simulink model "AFlutter"  (Simulink 7.7)
settings: Solver=FixedStepDiscrete  StartTime=0.0  StopTime=1000000  FixedStep=1  RelTol=1e-3
libraries: LookupModeling x68
settings Model: Creator=iris  LastModifiedBy=iris

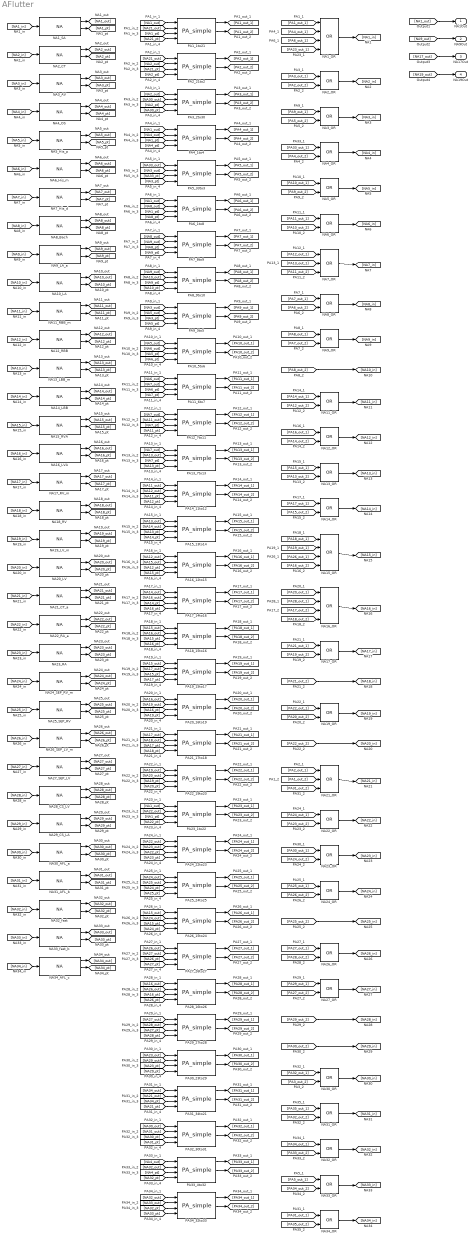
== system AFlutter ==
  NA10_LA : LookupModeling/NA  SystemSampleTime=-1  TERP_s_m=360  TERP_defs_m=360  TRRP_s_m=120  TRRP_def_m=120  Trest_s_m=9999  Trest_def_m=9999  Terp_min_m=150  Terp_max_m=360
  NA11_OR : Logic  Operator=OR  AllPortsSameDT=off  OutDataTypeStr=boolean
  NA11_RBB_m : LookupModeling/NA  SystemSampleTime=-1  TERP_s_m=440  TERP_defs_m=440  TRRP_s_m=120  TRRP_def_m=120  Trest_s_m=9999  Trest_def_m=9999  Terp_min_m=330  Terp_max_m=440
  NA12_OR : Logic  Operator=OR  AllPortsSameDT=off  OutDataTypeStr=boolean
  NA12_RBB : LookupModeling/NA  SystemSampleTime=-1  TERP_s_m=440  TERP_defs_m=440  TRRP_s_m=120  TRRP_def_m=120  Trest_s_m=9999  Trest_def_m=9999  Terp_min_m=330  Terp_max_m=440
  NA13_LBB_m : LookupModeling/NA  SystemSampleTime=-1  TERP_s_m=440  TERP_defs_m=440  TRRP_s_m=120  TRRP_def_m=120  Trest_s_m=9999  Trest_def_m=9999  Terp_min_m=330  Terp_max_m=440
  NA13_OR : Logic  Operator=OR  AllPortsSameDT=off  OutDataTypeStr=boolean
  NA14_LBB : LookupModeling/NA  SystemSampleTime=-1  TERP_s_m=440  TERP_defs_m=440  TRRP_s_m=120  TRRP_def_m=120  Trest_s_m=9999  Trest_def_m=9999  Terp_min_m=330  Terp_max_m=440
  NA14_OR : Logic  Operator=OR  AllPortsSameDT=off  OutDataTypeStr=boolean
  NA15_OR : Logic  Operator=OR  Inputs=4  AllPortsSameDT=off  OutDataTypeStr=boolean
  NA15_RVA : LookupModeling/NA  SystemSampleTime=-1  TERP_s_m=290  TERP_defs_m=290  TRRP_s_m=120  TRRP_def_m=120  Trest_s_m=9999  Trest_def_m=9999  Terp_min_m=180  Terp_max_m=290
  NA16_LVA : LookupModeling/NA  SystemSampleTime=-1  TERP_s_m=290  TERP_defs_m=290  TRRP_s_m=120  TRRP_def_m=120  Trest_s_m=9999  Trest_def_m=9999  Terp_min_m=180  Terp_max_m=290
  NA16_OR : Logic  Operator=OR  Inputs=4  AllPortsSameDT=off  OutDataTypeStr=boolean
  NA17_OR : Logic  Operator=OR  AllPortsSameDT=off  OutDataTypeStr=boolean
  NA17_RV_m : LookupModeling/NA  SystemSampleTime=-1  TERP_s_m=290  TERP_defs_m=290  TRRP_s_m=120  TRRP_def_m=120  Trest_s_m=9999  Trest_def_m=9999  Terp_min_m=180  Terp_max_m=290
  NA18_RV : LookupModeling/NA  SystemSampleTime=-1  TERP_s_m=290  TERP_defs_m=290  TRRP_s_m=120  TRRP_def_m=120  Trest_s_m=9999  Trest_def_m=9999  Terp_min_m=180  Terp_max_m=290
  NA19_LV_m : LookupModeling/NA  SystemSampleTime=-1  TERP_s_m=303  TERP_defs_m=290  TRRP_s_m=120  TRRP_def_m=120  Trest_s_m=9999  Trest_def_m=9999  Terp_min_m=180  Terp_max_m=290
  NA19_OR : Logic  Operator=OR  AllPortsSameDT=off  OutDataTypeStr=boolean
  NA1_OR : Logic  Operator=OR  Inputs=4  AllPortsSameDT=off  OutDataTypeStr=boolean
  NA1_SA : LookupModeling/NA  SystemSampleTime=-1  TERP_s_m=150  TERP_defs_m=150  TRRP_s_m=20  TRRP_def_m=20  Trest_s_m=500  Trest_def_m=700  Terp_min_m=150  Terp_max_m=300
  NA20_LV : LookupModeling/NA  SystemSampleTime=-1  TERP_s_m=290  TERP_defs_m=290  TRRP_s_m=120  TRRP_def_m=120  Trest_s_m=9999  Trest_def_m=9999  Terp_min_m=180  Terp_max_m=290
  NA21_CT_a : LookupModeling/NA  SystemSampleTime=-1  TERP_s_m=180  TERP_defs_m=180  TRRP_s_m=120  TRRP_def_m=120  Trest_s_m=9999  Trest_def_m=9999  Terp_min_m=150  Terp_max_m=200
  NA21_OR : Logic  Operator=OR  Inputs=3  AllPortsSameDT=off  OutDataTypeStr=boolean
  NA22_OR : Logic  Operator=OR  AllPortsSameDT=off  OutDataTypeStr=boolean
  NA22_RA_a : LookupModeling/NA  SystemSampleTime=-1  TERP_s_m=360  TERP_defs_m=360  TRRP_s_m=120  TRRP_def_m=120  Trest_s_m=9999  Trest_def_m=9999  Terp_min_m=150  Terp_max_m=360
  NA23_OR : Logic  Operator=OR  AllPortsSameDT=off  OutDataTypeStr=boolean
  NA23_RA : LookupModeling/NA  SystemSampleTime=-1  TERP_s_m=360  TERP_defs_m=360  TRRP_s_m=120  TRRP_def_m=120  Trest_s_m=9999  Trest_def_m=9999  Terp_min_m=150  Terp_max_m=360
  NA24_OR : Logic  Operator=OR  AllPortsSameDT=off  OutDataTypeStr=boolean
  NA24_SEP_RV_m : LookupModeling/NA  SystemSampleTime=-1  TERP_s_m=300  TERP_defs_m=300  TRRP_s_m=120  TRRP_def_m=120  Trest_s_m=9999  Trest_def_m=9999  Terp_min_m=150  Terp_max_m=300
  NA25_SEP_RV : LookupModeling/NA  SystemSampleTime=-1  TERP_s_m=300  TERP_defs_m=300  TRRP_s_m=120  TRRP_def_m=120  Trest_s_m=9999  Trest_def_m=9999  Terp_min_m=150  Terp_max_m=300
  NA26_OR : Logic  Operator=OR  AllPortsSameDT=off  OutDataTypeStr=boolean
  NA26_SEP_LV_m : LookupModeling/NA  SystemSampleTime=-1  TERP_s_m=300  TERP_defs_m=300  TRRP_s_m=120  TRRP_def_m=120  Trest_s_m=9999  Trest_def_m=9999  Terp_min_m=150  Terp_max_m=300
  NA27_OR : Logic  Operator=OR  AllPortsSameDT=off  OutDataTypeStr=boolean
  NA27_SEP_LV : LookupModeling/NA  SystemSampleTime=-1  TERP_s_m=300  TERP_defs_m=300  TRRP_s_m=120  TRRP_def_m=120  Trest_s_m=9999  Trest_def_m=9999  Terp_min_m=150  Terp_max_m=300
  NA28_CS_LV : LookupModeling/NA  SystemSampleTime=-1  TERP_s_m=300  TERP_defs_m=300  TRRP_s_m=120  TRRP_def_m=120  Trest_s_m=9999  Trest_def_m=9999  Terp_min_m=150  Terp_max_m=300
  NA29_CS_LA : LookupModeling/NA  SystemSampleTime=-1  TERP_s_m=300  TERP_defs_m=300  TRRP_s_m=120  TRRP_def_m=120  Trest_s_m=9999  Trest_def_m=9999  Terp_min_m=150  Terp_max_m=300
  NA2_CT : LookupModeling/NA  SystemSampleTime=-1  TERP_s_m=150  TERP_defs_m=150  TRRP_s_m=100  TRRP_def_m=100  Trest_s_m=9999  Trest_def_m=9999  Terp_min_m=50  Terp_max_m=150
  NA2_OR : Logic  Operator=OR  AllPortsSameDT=off  OutDataTypeStr=boolean
  NA30_AFL_a : LookupModeling/NA  SystemSampleTime=-1  TERP_s_m=150  TERP_defs_m=150  TRRP_s_m=100  TRRP_def_m=100  Trest_s_m=9999  Trest_def_m=9999  Terp_min_m=150  Terp_max_m=200
  NA30_OR : Logic  Operator=OR  AllPortsSameDT=off  OutDataTypeStr=boolean
  NA31_AFL_b : LookupModeling/NA  SystemSampleTime=-1  TERP_s_m=150  TERP_defs_m=150  TRRP_s_m=100  TRRP_def_m=100  Trest_s_m=9999  Trest_def_m=9999  Terp_min_m=150  Terp_max_m=200
  NA31_OR : Logic  Operator=OR  AllPortsSameDT=off  OutDataTypeStr=boolean
  NA32_OR : Logic  Operator=OR  AllPortsSameDT=off  OutDataTypeStr=boolean
  NA32_fast : LookupModeling/NA  SystemSampleTime=-1  TERP_s_m=380  TERP_defs_m=380  TRRP_s_m=10  TRRP_def_m=10  Trest_s_m=9999  Trest_def_m=9999  Terp_min_m=500  Terp_max_m=380
  NA33_OR : Logic  Operator=OR  AllPortsSameDT=off  OutDataTypeStr=boolean
  NA33_fast_b : LookupModeling/NA  SystemSampleTime=-1  TERP_s_m=380  TERP_defs_m=380  TRRP_s_m=10  TRRP_def_m=10  Trest_s_m=9999  Trest_def_m=9999  Terp_min_m=500  Terp_max_m=380
  NA34_AFL_c : LookupModeling/NA  SystemSampleTime=-1  TERP_s_m=150  TERP_defs_m=150  TRRP_s_m=100  TRRP_def_m=100  Trest_s_m=9999  Trest_def_m=9999  Terp_min_m=150  Terp_max_m=200
  NA34_OR : Logic  Operator=OR  AllPortsSameDT=off  OutDataTypeStr=boolean
  NA3_AV : LookupModeling/NA  SystemSampleTime=-1  TERP_s_m=230  TERP_defs_m=230  TRRP_s_m=250  TRRP_def_m=250  Trest_s_m=9999  Trest_def_m=9999  Terp_min_m=350  Terp_max_m=230
  NA3_OR : Logic  Operator=OR  AllPortsSameDT=off  OutDataTypeStr=boolean
  NA4_OR : Logic  Operator=OR  AllPortsSameDT=off  OutDataTypeStr=boolean
  NA4_OS : LookupModeling/NA  SystemSampleTime=-1  TERP_s_m=200  TERP_defs_m=200  TRRP_s_m=120  TRRP_def_m=120  Trest_s_m=9999  Trest_def_m=9999  Terp_min_m=100  Terp_max_m=200
  NA5_His_p : LookupModeling/NA  SystemSampleTime=-1  TERP_s_m=440  TERP_defs_m=440  TRRP_s_m=120  TRRP_def_m=120  Trest_s_m=9999  Trest_def_m=9999  Terp_min_m=330  Terp_max_m=440
  NA5_OR : Logic  Operator=OR  AllPortsSameDT=off  OutDataTypeStr=boolean
  NA6_His_m : LookupModeling/NA  SystemSampleTime=-1  TERP_s_m=440  TERP_defs_m=440  TRRP_s_m=120  TRRP_def_m=120  Trest_s_m=9999  Trest_def_m=9999  Terp_min_m=330  Terp_max_m=440
  NA6_OR : Logic  Operator=OR  AllPortsSameDT=off  OutDataTypeStr=boolean
  NA7_His_d : LookupModeling/NA  SystemSampleTime=-1  TERP_s_m=440  TERP_defs_m=440  TRRP_s_m=120  TRRP_def_m=120  Trest_s_m=9999  Trest_def_m=9999  Terp_min_m=330  Terp_max_m=440
  NA7_OR : Logic  Operator=OR  Inputs=3  AllPortsSameDT=off  OutDataTypeStr=boolean
  NA8_Bach : LookupModeling/NA  SystemSampleTime=-1  TERP_s_m=360  TERP_defs_m=360  TRRP_s_m=120  TRRP_def_m=120  Trest_s_m=9999  Trest_def_m=9999  Terp_min_m=150  Terp_max_m=360
  NA8_OR : Logic  Operator=OR  AllPortsSameDT=off  OutDataTypeStr=boolean
  NA9_LA_a : LookupModeling/NA  SystemSampleTime=-1  TERP_s_m=360  TERP_defs_m=360  TRRP_s_m=120  TRRP_def_m=120  Trest_s_m=9999  Trest_def_m=9999  Terp_min_m=150  Terp_max_m=360
  NA9_OR : Logic  Operator=OR  AllPortsSameDT=off  OutDataTypeStr=boolean
  PA10_5to6 : LookupModeling/PA_simple  SystemSampleTime=-1  min_path_par_m=16  bck_param_m=16  forw_param_m=16
  PA11_6to7 : LookupModeling/PA_simple  SystemSampleTime=-1  min_path_par_m=19  bck_param_m=20  forw_param_m=20
  PA12_7to11 : LookupModeling/PA_simple  SystemSampleTime=-1  min_path_par_m=36  bck_param_m=36  forw_param_m=36
  PA13_7to13 : LookupModeling/PA_simple  SystemSampleTime=-1  min_path_par_m=37  bck_param_m=37  forw_param_m=37
  PA14_11to12 : LookupModeling/PA_simple  SystemSampleTime=-1  min_path_par_m=20  bck_param_m=20  forw_param_m=20
  PA15_13to14 : LookupModeling/PA_simple  SystemSampleTime=-1  min_path_par_m=19  bck_param_m=20  forw_param_m=20
  PA16_12to15 : LookupModeling/PA_simple  SystemSampleTime=-1  min_path_par_m=18  bck_param_m=18  forw_param_m=18
  PA17_14to16 : LookupModeling/PA_simple  SystemSampleTime=-1  min_path_par_m=18  bck_param_m=19  forw_param_m=19
  PA18_15to16 : LookupModeling/PA_simple  SystemSampleTime=-1  min_path_par_m=17  bck_param_m=17  forw_param_m=17
  PA19_15to17 : LookupModeling/PA_simple  SystemSampleTime=-1  min_path_par_m=19  bck_param_m=20  forw_param_m=20
  PA1_1to21 : LookupModeling/PA_simple  SystemSampleTime=-1  min_path_par_m=57  bck_param_m=57  forw_param_m=57
  PA20_16to19 : LookupModeling/PA_simple  SystemSampleTime=-1  min_path_par_m=20  bck_param_m=20  forw_param_m=20
  PA21_17to18 : LookupModeling/PA_simple  SystemSampleTime=-1  min_path_par_m=19  bck_param_m=20  forw_param_m=20
  PA22_19to20 : LookupModeling/PA_simple  SystemSampleTime=-1  min_path_par_m=20  bck_param_m=20  forw_param_m=20
  PA23_1to22 : LookupModeling/PA_simple  SystemSampleTime=-1  min_path_par_m=40  bck_param_m=40  forw_param_m=40
  PA24_22to23 : LookupModeling/PA_simple  SystemSampleTime=-1  min_path_par_m=35  bck_param_m=35  forw_param_m=35
  PA25_24to25 : LookupModeling/PA_simple  SystemSampleTime=-1  min_path_par_m=56  bck_param_m=56  forw_param_m=56
  PA26_15to24 : LookupModeling/PA_simple  SystemSampleTime=-1  min_path_par_m=56  bck_param_m=57  forw_param_m=57
  PA27_26to27 : LookupModeling/PA_simple  SystemSampleTime=-1  min_path_par_m=52  bck_param_m=52  forw_param_m=52
  PA28_16to26 : LookupModeling/PA_simple  SystemSampleTime=-1  min_path_par_m=47  bck_param_m=47  forw_param_m=47
  PA29_27to28 : LookupModeling/PA_simple  SystemSampleTime=-1  min_path_par_m=39  bck_param_m=39  forw_param_m=39
  PA2_21to2 : LookupModeling/PA_simple  SystemSampleTime=-1  min_path_par_m=28  bck_param_m=28  forw_param_m=28
  PA30_23to29 : LookupModeling/PA_simple  SystemSampleTime=-1  min_path_par_m=59  bck_param_m=59  forw_param_m=59
  PA31_34to21 : LookupModeling/PA_simple  SystemSampleTime=-1  min_path_par_m=42  bck_param_m=42  forw_param_m=42
  PA32_30to31 : LookupModeling/PA_simple  SystemSampleTime=-1  min_path_par_m=25  bck_param_m=25  forw_param_m=25
  PA33_4to32 : LookupModeling/PA_simple  SystemSampleTime=-1  min_path_par_m=10  bck_param_m=10  forw_param_m=10
  PA34_32to33 : LookupModeling/PA_simple  SystemSampleTime=-1  min_path_par_m=7  bck_param_m=7  forw_param_m=7
  PA3_2to30 : LookupModeling/PA_simple  SystemSampleTime=-1  min_path_par_m=96  bck_param_m=96  forw_param_m=96
  PA4_1to4 : LookupModeling/PA_simple  SystemSampleTime=-1  min_path_par_m=44  bck_param_m=44  forw_param_m=44
  PA5_33to3 : LookupModeling/PA_simple  SystemSampleTime=-1  min_path_par_m=14  bck_param_m=14  forw_param_m=14
  PA6_1to8 : LookupModeling/PA_simple  SystemSampleTime=-1  min_path_par_m=40  bck_param_m=40  forw_param_m=40
  PA7_8to9 : LookupModeling/PA_simple  SystemSampleTime=-1  min_path_par_m=68  bck_param_m=68  forw_param_m=68
  PA8_9to10 : LookupModeling/PA_simple  SystemSampleTime=-1  min_path_par_m=33  bck_param_m=35  forw_param_m=35
  PA9_3to5 : LookupModeling/PA_simple  SystemSampleTime=-1  min_path_par_m=47  bck_param_m=47  forw_param_m=47
  NA1Out : Outport
  NA9Out : Outport  Port=2
  NA17Out : Outport  Port=3
  NA19Out : Outport  Port=4
  wires:
  NA1_SA/1 -> [NA1_out]
  NA1_SA/3 -> [NA1_pt]
  [NA1_in] -> NA1_SA/1
  NA1_OR/1 -> [NA1_in]
  [PA1_out_1] -> NA1_OR/1
  [PA4_out_1] -> NA1_OR/2
  [PA6_out_1] -> NA1_OR/3
  [PA23_out_1] -> NA1_OR/4
  NA2_CT/1 -> [NA2_out]
  NA2_CT/3 -> [NA2_pt]
  [NA2_in] -> NA2_CT/1
  NA2_OR/1 -> [NA2_in]
  [PA3_out_1] -> NA2_OR/1
  [PA2_out_2] -> NA2_OR/2
  NA3_AV/1 -> [NA3_out]
  NA3_AV/3 -> [NA3_pt]
  [NA3_in] -> NA3_AV/1
  NA3_OR/1 -> [NA3_in]
  [PA9_out_1] -> NA3_OR/1
  [PA5_out_2] -> NA3_OR/2
  NA4_OS/1 -> [NA4_out]
  NA4_OS/3 -> [NA4_pt]
  [NA4_in] -> NA4_OS/1
  NA4_OR/1 -> [NA4_in]
  [PA33_out_1] -> NA4_OR/1
  [PA4_out_2] -> NA4_OR/2
  NA5_His_p/1 -> [NA5_out]
  NA5_His_p/3 -> [NA5_pt]
  [NA5_in] -> NA5_His_p/1
  NA5_OR/1 -> [NA5_in]
  [PA10_out_1] -> NA5_OR/1
  [PA9_out_2] -> NA5_OR/2
  NA6_His_m/1 -> [NA6_out]
  NA6_His_m/3 -> [NA6_pt]
  [NA6_in] -> NA6_His_m/1
  NA6_OR/1 -> [NA6_in]
  [PA11_out_1] -> NA6_OR/1
  [PA10_out_2] -> NA6_OR/2
  NA7_His_d/1 -> [NA7_out]
  NA7_His_d/3 -> [NA7_pt]
  [NA7_in] -> NA7_His_d/1
  NA7_OR/1 -> [NA7_in]
  [PA12_out_1] -> NA7_OR/1
  [PA13_out_1] -> NA7_OR/2
  [PA11_out_2] -> NA7_OR/3
  NA8_Bach/1 -> [NA8_out]
  NA8_Bach/3 -> [NA8_pt]
  [NA8_in] -> NA8_Bach/1
  NA8_OR/1 -> [NA8_in]
  [PA7_out_1] -> NA8_OR/1
  [PA6_out_2] -> NA8_OR/2
  NA9_LA_a/1 -> [NA9_out]
  NA9_LA_a/3 -> [NA9_pt]
  [NA9_in] -> NA9_LA_a/1
  NA9_OR/1 -> [NA9_in]
  [PA8_out_1] -> NA9_OR/1
  [PA7_out_2] -> NA9_OR/2
  NA10_LA/1 -> [NA10_out]
  NA10_LA/3 -> [NA10_pt]
  [NA10_in] -> NA10_LA/1
  [PA8_out_2] -> [NA10_in]
  NA11_RBB_m/1 -> [NA11_out]
  NA11_RBB_m/3 -> [NA11_pt]
  [NA11_in] -> NA11_RBB_m/1
  NA11_OR/1 -> [NA11_in]
  [PA14_out_1] -> NA11_OR/1
  [PA12_out_2] -> NA11_OR/2
  NA12_RBB/1 -> [NA12_out]
  NA12_RBB/3 -> [NA12_pt]
  [NA12_in] -> NA12_RBB/1
  NA12_OR/1 -> [NA12_in]
  [PA16_out_1] -> NA12_OR/1
  [PA14_out_2] -> NA12_OR/2
  NA13_LBB_m/1 -> [NA13_out]
  NA13_LBB_m/3 -> [NA13_pt]
  [NA13_in] -> NA13_LBB_m/1
  NA13_OR/1 -> [NA13_in]
  [PA15_out_1] -> NA13_OR/1
  [PA13_out_2] -> NA13_OR/2
  NA14_LBB/1 -> [NA14_out]
  NA14_LBB/3 -> [NA14_pt]
  [NA14_in] -> NA14_LBB/1
  NA14_OR/1 -> [NA14_in]
  [PA17_out_1] -> NA14_OR/1
  [PA15_out_2] -> NA14_OR/2
  NA15_RVA/1 -> [NA15_out]
  NA15_RVA/3 -> [NA15_pt]
  [NA15_in] -> NA15_RVA/1
  NA15_OR/1 -> [NA15_in]
  [PA18_out_1] -> NA15_OR/1
  [PA19_out_1] -> NA15_OR/2
  [PA26_out_1] -> NA15_OR/3
  [PA16_out_2] -> NA15_OR/4
  NA16_LVA/1 -> [NA16_out]
  NA16_LVA/3 -> [NA16_pt]
  [NA16_in] -> NA16_LVA/1
  NA16_OR/1 -> [NA16_in]
  [PA20_out_1] -> NA16_OR/1
  [PA28_out_1] -> NA16_OR/2
  [PA17_out_2] -> NA16_OR/3
  [PA18_out_2] -> NA16_OR/4
  NA17_RV_m/1 -> [NA17_out]
  NA17_RV_m/3 -> [NA17_pt]
  [NA17_in] -> NA17_RV_m/1
  NA17_OR/1 -> [NA17_in]
  [PA21_out_1] -> NA17_OR/1
  [PA19_out_2] -> NA17_OR/2
  NA18_RV/1 -> [NA18_out]
  NA18_RV/3 -> [NA18_pt]
  [NA18_in] -> NA18_RV/1
  [PA21_out_2] -> [NA18_in]
  NA19_LV_m/1 -> [NA19_out]
  NA19_LV_m/3 -> [NA19_pt]
  [NA19_in] -> NA19_LV_m/1
  NA19_OR/1 -> [NA19_in]
  [PA22_out_1] -> NA19_OR/1
  [PA20_out_2] -> NA19_OR/2
  NA20_LV/1 -> [NA20_out]
  NA20_LV/3 -> [NA20_pt]
  [NA20_in] -> NA20_LV/1
  [PA22_out_2] -> [NA20_in]
  NA21_CT_a/1 -> [NA21_out]
  NA21_CT_a/3 -> [NA21_pt]
  [NA21_in] -> NA21_CT_a/1
  NA21_OR/1 -> [NA21_in]
  [PA2_out_1] -> NA21_OR/1
  [PA1_out_2] -> NA21_OR/2
  [PA31_out_2] -> NA21_OR/3
  NA22_RA_a/1 -> [NA22_out]
  NA22_RA_a/3 -> [NA22_pt]
  [NA22_in] -> NA22_RA_a/1
  NA22_OR/1 -> [NA22_in]
  [PA24_out_1] -> NA22_OR/1
  [PA23_out_2] -> NA22_OR/2
  NA23_RA/1 -> [NA23_out]
  NA23_RA/3 -> [NA23_pt]
  [NA23_in] -> NA23_RA/1
  NA23_OR/1 -> [NA23_in]
  [PA30_out_1] -> NA23_OR/1
  [PA24_out_2] -> NA23_OR/2
  NA24_SEP_RV_m/1 -> [NA24_out]
  NA24_SEP_RV_m/3 -> [NA24_pt]
  [NA24_in] -> NA24_SEP_RV_m/1
  NA24_OR/1 -> [NA24_in]
  [PA25_out_1] -> NA24_OR/1
  [PA26_out_2] -> NA24_OR/2
  NA25_SEP_RV/1 -> [NA25_out]
  NA25_SEP_RV/3 -> [NA25_pt]
  [NA25_in] -> NA25_SEP_RV/1
  [PA25_out_2] -> [NA25_in]
  NA26_SEP_LV_m/1 -> [NA26_out]
  NA26_SEP_LV_m/3 -> [NA26_pt]
  [NA26_in] -> NA26_SEP_LV_m/1
  NA26_OR/1 -> [NA26_in]
  [PA27_out_1] -> NA26_OR/1
  [PA28_out_2] -> NA26_OR/2
  NA27_SEP_LV/1 -> [NA27_out]
  NA27_SEP_LV/3 -> [NA27_pt]
  [NA27_in] -> NA27_SEP_LV/1
  NA27_OR/1 -> [NA27_in]
  [PA29_out_1] -> NA27_OR/1
  [PA27_out_2] -> NA27_OR/2
  NA28_CS_LV/1 -> [NA28_out]
  NA28_CS_LV/3 -> [NA28_pt]
  [NA28_in] -> NA28_CS_LV/1
  [PA29_out_2] -> [NA28_in]
  NA29_CS_LA/1 -> [NA29_out]
  NA29_CS_LA/3 -> [NA29_pt]
  [NA29_in] -> NA29_CS_LA/1
  [PA30_out_2] -> [NA29_in]
  NA30_AFL_a/1 -> [NA30_out]
  NA30_AFL_a/3 -> [NA30_pt]
  [NA30_in] -> NA30_AFL_a/1
  NA30_OR/1 -> [NA30_in]
  [PA32_out_1] -> NA30_OR/1
  [PA3_out_2] -> NA30_OR/2
  NA31_AFL_b/1 -> [NA31_out]
  NA31_AFL_b/3 -> [NA31_pt]
  [NA31_in] -> NA31_AFL_b/1
  NA31_OR/1 -> [NA31_in]
  [PA35_out_1] -> NA31_OR/1
  [PA32_out_2] -> NA31_OR/2
  NA32_fast/1 -> [NA32_out]
  NA32_fast/3 -> [NA32_pt]
  [NA32_in] -> NA32_fast/1
  NA32_OR/1 -> [NA32_in]
  [PA34_out_1] -> NA32_OR/1
  [PA33_out_2] -> NA32_OR/2
  NA33_fast_b/1 -> [NA33_out]
  NA33_fast_b/3 -> [NA33_pt]
  [NA33_in] -> NA33_fast_b/1
  NA33_OR/1 -> [NA33_in]
  [PA5_out_1] -> NA33_OR/1
  [PA34_out_2] -> NA33_OR/2
  NA34_AFL_c/1 -> [NA34_out]
  NA34_AFL_c/3 -> [NA34_pt]
  [NA34_in] -> NA34_AFL_c/1
  NA34_OR/1 -> [NA34_in]
  [PA31_out_1] -> NA34_OR/1
  [PA35_out_2] -> NA34_OR/2
  PA1_1to21/1 -> [PA1_out_1]
  PA1_1to21/2 -> [PA1_out_2]
  [NA1_out] -> PA1_1to21/1
  [NA21_out] -> PA1_1to21/2
  [NA1_pt] -> PA1_1to21/3
  [NA21_pt] -> PA1_1to21/4
  PA2_21to2/1 -> [PA2_out_1]
  PA2_21to2/2 -> [PA2_out_2]
  [NA21_out] -> PA2_21to2/1
  [NA2_out] -> PA2_21to2/2
  [NA21_pt] -> PA2_21to2/3
  [NA2_pt] -> PA2_21to2/4
  PA3_2to30/1 -> [PA3_out_1]
  PA3_2to30/2 -> [PA3_out_2]
  [NA2_out] -> PA3_2to30/1
  [NA30_out] -> PA3_2to30/2
  [NA2_pt] -> PA3_2to30/3
  [NA30_pt] -> PA3_2to30/4
  PA4_1to4/1 -> [PA4_out_1]
  PA4_1to4/2 -> [PA4_out_2]
  [NA1_out] -> PA4_1to4/1
  [NA4_out] -> PA4_1to4/2
  [NA1_pt] -> PA4_1to4/3
  [NA4_pt] -> PA4_1to4/4
  PA5_33to3/1 -> [PA5_out_1]
  PA5_33to3/2 -> [PA5_out_2]
  [NA33_out] -> PA5_33to3/1
  [NA3_out] -> PA5_33to3/2
  [NA33_pt] -> PA5_33to3/3
  [NA3_pt] -> PA5_33to3/4
  PA6_1to8/1 -> [PA6_out_1]
  PA6_1to8/2 -> [PA6_out_2]
  [NA1_out] -> PA6_1to8/1
  [NA8_out] -> PA6_1to8/2
  [NA1_pt] -> PA6_1to8/3
  [NA8_pt] -> PA6_1to8/4
  PA7_8to9/1 -> [PA7_out_1]
  PA7_8to9/2 -> [PA7_out_2]
  [NA8_out] -> PA7_8to9/1
  [NA9_out] -> PA7_8to9/2
  [NA8_pt] -> PA7_8to9/3
  [NA9_pt] -> PA7_8to9/4
  PA8_9to10/1 -> [PA8_out_1]
  PA8_9to10/2 -> [PA8_out_2]
  [NA9_out] -> PA8_9to10/1
  [NA10_out] -> PA8_9to10/2
  [NA9_pt] -> PA8_9to10/3
  [NA10_pt] -> PA8_9to10/4
  PA9_3to5/1 -> [PA9_out_1]
  PA9_3to5/2 -> [PA9_out_2]
  [NA3_out] -> PA9_3to5/1
  [NA5_out] -> PA9_3to5/2
  [NA3_pt] -> PA9_3to5/3
  [NA5_pt] -> PA9_3to5/4
  PA10_5to6/1 -> [PA10_out_1]
  PA10_5to6/2 -> [PA10_out_2]
  [NA5_out] -> PA10_5to6/1
  [NA6_out] -> PA10_5to6/2
  [NA5_pt] -> PA10_5to6/3
  [NA6_pt] -> PA10_5to6/4
  PA11_6to7/1 -> [PA11_out_1]
  PA11_6to7/2 -> [PA11_out_2]
  [NA6_out] -> PA11_6to7/1
  [NA7_out] -> PA11_6to7/2
  [NA6_pt] -> PA11_6to7/3
  [NA7_pt] -> PA11_6to7/4
  PA12_7to11/1 -> [PA12_out_1]
  PA12_7to11/2 -> [PA12_out_2]
  [NA7_out] -> PA12_7to11/1
  [NA11_out] -> PA12_7to11/2
  [NA7_pt] -> PA12_7to11/3
  [NA11_pt] -> PA12_7to11/4
  PA13_7to13/1 -> [PA13_out_1]
  PA13_7to13/2 -> [PA13_out_2]
  [NA7_out] -> PA13_7to13/1
  [NA13_out] -> PA13_7to13/2
  [NA7_pt] -> PA13_7to13/3
  [NA13_pt] -> PA13_7to13/4
  PA14_11to12/1 -> [PA14_out_1]
  PA14_11to12/2 -> [PA14_out_2]
  [NA11_out] -> PA14_11to12/1
  [NA12_out] -> PA14_11to12/2
  [NA11_pt] -> PA14_11to12/3
  [NA12_pt] -> PA14_11to12/4
  PA15_13to14/1 -> [PA15_out_1]
  PA15_13to14/2 -> [PA15_out_2]
  [NA13_out] -> PA15_13to14/1
  [NA14_out] -> PA15_13to14/2
  [NA13_pt] -> PA15_13to14/3
  [NA14_pt] -> PA15_13to14/4
  PA16_12to15/1 -> [PA16_out_1]
  PA16_12to15/2 -> [PA16_out_2]
  [NA12_out] -> PA16_12to15/1
  [NA15_out] -> PA16_12to15/2
  [NA12_pt] -> PA16_12to15/3
  [NA15_pt] -> PA16_12to15/4
  PA17_14to16/1 -> [PA17_out_1]
  PA17_14to16/2 -> [PA17_out_2]
  [NA14_out] -> PA17_14to16/1
  [NA16_out] -> PA17_14to16/2
  [NA14_pt] -> PA17_14to16/3
  [NA16_pt] -> PA17_14to16/4
  PA18_15to16/1 -> [PA18_out_1]
  PA18_15to16/2 -> [PA18_out_2]
  [NA15_out] -> PA18_15to16/1
  [NA16_out] -> PA18_15to16/2
  [NA15_pt] -> PA18_15to16/3
  [NA16_pt] -> PA18_15to16/4
  PA19_15to17/1 -> [PA19_out_1]
  PA19_15to17/2 -> [PA19_out_2]
  [NA15_out] -> PA19_15to17/1
  [NA17_out] -> PA19_15to17/2
  [NA15_pt] -> PA19_15to17/3
  [NA17_pt] -> PA19_15to17/4
  PA20_16to19/1 -> [PA20_out_1]
  PA20_16to19/2 -> [PA20_out_2]
  [NA16_out] -> PA20_16to19/1
  [NA19_out] -> PA20_16to19/2
  [NA16_pt] -> PA20_16to19/3
  [NA19_pt] -> PA20_16to19/4
  PA21_17to18/1 -> [PA21_out_1]
  PA21_17to18/2 -> [PA21_out_2]
  [NA17_out] -> PA21_17to18/1
  [NA18_out] -> PA21_17to18/2
  [NA17_pt] -> PA21_17to18/3
  [NA18_pt] -> PA21_17to18/4
  PA22_19to20/1 -> [PA22_out_1]
  PA22_19to20/2 -> [PA22_out_2]
  [NA19_out] -> PA22_19to20/1
  [NA20_out] -> PA22_19to20/2
  [NA19_pt] -> PA22_19to20/3
  [NA20_pt] -> PA22_19to20/4
  PA23_1to22/1 -> [PA23_out_1]
  PA23_1to22/2 -> [PA23_out_2]
  [NA1_out] -> PA23_1to22/1
  [NA22_out] -> PA23_1to22/2
  [NA1_pt] -> PA23_1to22/3
  [NA22_pt] -> PA23_1to22/4
  PA24_22to23/1 -> [PA24_out_1]
  PA24_22to23/2 -> [PA24_out_2]
  [NA22_out] -> PA24_22to23/1
  [NA23_out] -> PA24_22to23/2
  [NA22_pt] -> PA24_22to23/3
  [NA23_pt] -> PA24_22to23/4
  PA25_24to25/1 -> [PA25_out_1]
  PA25_24to25/2 -> [PA25_out_2]
  [NA24_out] -> PA25_24to25/1
  [NA25_out] -> PA25_24to25/2
  [NA24_pt] -> PA25_24to25/3
  [NA25_pt] -> PA25_24to25/4
  PA26_15to24/1 -> [PA26_out_1]
  PA26_15to24/2 -> [PA26_out_2]
  [NA15_out] -> PA26_15to24/1
  [NA24_out] -> PA26_15to24/2
  [NA15_pt] -> PA26_15to24/3
  [NA24_pt] -> PA26_15to24/4
  PA27_26to27/1 -> [PA27_out_1]
  PA27_26to27/2 -> [PA27_out_2]
  [NA26_out] -> PA27_26to27/1
  [NA27_out] -> PA27_26to27/2
  [NA26_pt] -> PA27_26to27/3
  [NA27_pt] -> PA27_26to27/4
  PA28_16to26/1 -> [PA28_out_1]
  PA28_16to26/2 -> [PA28_out_2]
  [NA16_out] -> PA28_16to26/1
  [NA26_out] -> PA28_16to26/2
  [NA16_pt] -> PA28_16to26/3
  [NA26_pt] -> PA28_16to26/4
  PA29_27to28/1 -> [PA29_out_1]
  PA29_27to28/2 -> [PA29_out_2]
  [NA27_out] -> PA29_27to28/1
  [NA28_out] -> PA29_27to28/2
  [NA27_pt] -> PA29_27to28/3
  [NA28_pt] -> PA29_27to28/4
  PA30_23to29/1 -> [PA30_out_1]
  PA30_23to29/2 -> [PA30_out_2]
  [NA23_out] -> PA30_23to29/1
  [NA29_out] -> PA30_23to29/2
  [NA23_pt] -> PA30_23to29/3
  [NA29_pt] -> PA30_23to29/4
  PA31_34to21/1 -> [PA31_out_1]
  PA31_34to21/2 -> [PA31_out_2]
  [NA34_out] -> PA31_34to21/1
  [NA21_out] -> PA31_34to21/2
  [NA34_pt] -> PA31_34to21/3
  [NA21_pt] -> PA31_34to21/4
  PA32_30to31/1 -> [PA32_out_1]
  PA32_30to31/2 -> [PA32_out_2]
  [NA30_out] -> PA32_30to31/1
  [NA31_out] -> PA32_30to31/2
  [NA30_pt] -> PA32_30to31/3
  [NA31_pt] -> PA32_30to31/4
  PA33_4to32/1 -> [PA33_out_1]
  PA33_4to32/2 -> [PA33_out_2]
  [NA4_out] -> PA33_4to32/1
  [NA32_out] -> PA33_4to32/2
  [NA4_pt] -> PA33_4to32/3
  [NA32_pt] -> PA33_4to32/4
  PA34_32to33/1 -> [PA34_out_1]
  PA34_32to33/2 -> [PA34_out_2]
  [NA32_out] -> PA34_32to33/1
  [NA33_out] -> PA34_32to33/2
  [NA32_pt] -> PA34_32to33/3
  [NA33_pt] -> PA34_32to33/4
  [NA1_out] -> NA1Out/1
  [NA9_out] -> NA9Out/1
  [NA17_out] -> NA17Out/1
  [NA19_out] -> NA19Out/1
